simulink model "Simple 64-bit ALU"  (R2015b)
settings: Solver=FixedStepDiscrete  SolverMode=SingleTasking  StartTime=0.0  StopTime=10.0  RelTol=1e-3
model workspace (MATLAB code in the model file):
  | A=[5 3];
  | B=[5 4];
  | C=[5 1];
libraries: shlslibv1 x11
settings Model: synDspstartup=OK  Creator=sjparekh  LastModifiedBy=sjparekh
settings DataIOCC: SaveOutput=off  SignalLogging=off  SaveTime=off
settings OptimizationCC: DefaultParameterBehavior=Inlined
settings DebuggingCC: AlgebraicLoopMsg=error

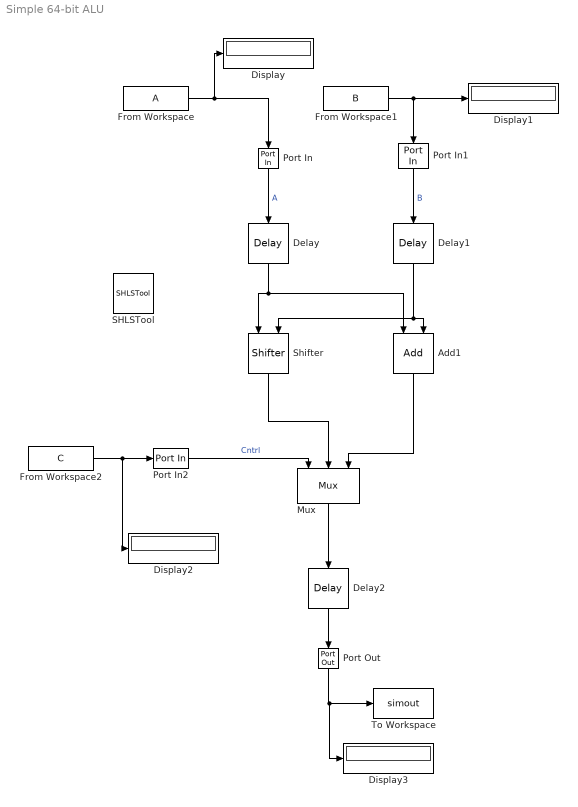
== system Simple 64-bit ALU ==
  Add1 : shlslibv1/Math Functions/Add  syn_add_opr=++  syn_out_f=Full Precision  syn_out_wl=16  syn_out_fl=8  syn_out_dt=signed  syn_out_sat=off  syn_out_rnd=Floor (Truncate)  synBlockType=primitive  synLatency=0  synBlockId=96  syn_sum_of_rows=off  syn_inh_port=off  syn_inh_st=off  syn_inh_stf=1  syn_en_pipe=off  syn_pipe_stg=syn_max_pipeline  syn_flow_ctrl=off
  Delay : shlslibv1/Memories/Delay  syn_delay_val=1  synBlockType=primitive  synLatency=1  synBlockId=104
  Delay1 : shlslibv1/Memories/Delay  syn_delay_val=1  synBlockType=primitive  synLatency=1  synBlockId=104
  Delay2 : shlslibv1/Memories/Delay  syn_delay_val=1  synBlockType=primitive  synLatency=1  synBlockId=104
  Display{,1..3} (4 alike) : Display
  From Workspace : FromWorkspace  VariableName=A  SampleTime=0
  From Workspace1 : FromWorkspace  VariableName=B  SampleTime=0
  From Workspace2 : FromWorkspace  VariableName=C  SampleTime=0
  Mux : shlslibv1/Signal Operations/Mux  syn_in_nb=2  syn_out_f=Full Precision  syn_out_wl=16  syn_out_fl=8  syn_out_dt=signed  syn_en_se=off  synBlockType=primitive  synLatency=0  synBlockId=16
  Port In : shlslibv1/Ports & Subsystems/Port In  syn_out_wl=64  syn_out_fl=0  syn_out_dt=signed  syn_out_st=1/20e6  syn_capture=on  syn_register=on  syn_out_sat=off  syn_out_rnd=on  synBlockType=port  synLatency=1  synBlockId=0
  Port In1 : shlslibv1/Ports & Subsystems/Port In  syn_out_wl=64  syn_out_fl=0  syn_out_dt=signed  syn_out_st=1/20e6  syn_capture=on  syn_register=on  syn_out_sat=off  syn_out_rnd=on  synBlockType=port  synLatency=1  synBlockId=0
  Port In2 : shlslibv1/Ports & Subsystems/Port In  syn_out_wl=64  syn_out_fl=0  syn_out_dt=signed  syn_out_st=1/20e6  syn_capture=on  syn_register=on  syn_out_sat=off  syn_out_rnd=on  synBlockType=port  synLatency=1  synBlockId=0
  Port Out : shlslibv1/Ports & Subsystems/Port Out  syn_capture=on  syn_register=on  synBlockType=port  synLatency=1  synBlockId=1
  SHLSTool : shlslibv1/SHLSTool  synBlockType=tool  syn_dsp_mode=FPGA
  Shifter : shlslibv1/Math Functions/Shifter  syn_shifter_opr=<<  syn_out_f=Automatic  syn_out_wl=16  syn_out_fl=8  syn_out_dt=signed  synBlockType=primitive  synLatency=0  synBlockId=12
  To Workspace : ToWorkspace  VariableName=simout  SaveFormat=Timeseries  SampleTime=-1
  wires:
  Delay/1 -> Add1/1, Shifter/1
  Delay1/1 -> Add1/2, Shifter/2
  Add1/1 -> Mux/3
  Shifter/1 -> Mux/2
  Port In2/1 -> Mux/1  "Cntrl"
  Mux/1 -> Delay2/1
  Delay2/1 -> Port Out/1
  Port In/1 -> Delay/1  "A"
  Port In1/1 -> Delay1/1  "B"
  From Workspace/1 -> Display/1, Port In/1
  From Workspace1/1 -> Display1/1, Port In1/1
  From Workspace2/1 -> Display2/1, Port In2/1
  Port Out/1 -> Display3/1, To Workspace/1
